simulink model "Fixed_Velocity_Fixed_Delta_TruckLab_A1"  (R2025b)
settings: Solver=ode4  StartTime=0  StopTime=130  FixedStep=1/120  RelTol=1e-3
undefined symbols (not defined in the file or in its folder): getRigidBodyPose, twist
libraries: simulink_extras x3, ros2lib x2
settings Model: Creator=20212285  LastModifiedBy=koenscholten
settings SolverCC: AlgebraicLoopSolver=LineSearch
settings DataIOCC: ReturnWorkspaceOutputsName=s
settings OptimizationCC: EnhancedBackFolding=on  PassReuseOutputArgsAs=Individual arguments  ZeroExternalMemoryAtStartup=off  ZeroInternalMemoryAtStartup=off  MaxStackSize=64  OptimizeBlockOrder=speed  DifferentSizesBufferReuse=on  OptimizationCustomize=off  EfficientTunableParamExpr=on
settings DebuggingCC: ParameterTunabilityLossMsg=error  UnconnectedInputMsg=warning  UnconnectedOutputMsg=warning  UnconnectedLineMsg=warning
settings ModelReferenceCC: EnableRefExpFcnMdlSchedulingChecks=on
settings SFSimCC: MATLABDynamicMemAlloc=off  SimTargetLang=C++  SimDLTargetLibrary=mkl-dnn
settings RTWCC: SystemTargetFile=ert.tlc  HardwareBoard=Robot Operating System 2 (ROS 2)  TLCOptions="-aInlineSetEventsForThisBaseRateFcn=TLC_FALSE -aSuppressMultiTaskScheduler=TLC_FALSE  -aRateBasedStepFcn=0"  TemplateMakefile=ert_default_tmf  Toolchain=Colcon Tools  TargetLang=C++  GPUComputeCapability=3.5  Description=Embedded Coder
settings CodeAppCC: ForceParamTrailComments=on  IgnoreCustomStorageClasses=off  OperatorAnnotations=on  SimulinkDataObjDesc=on  SFDataObjDesc=on  InsertBlockDesc=on
settings ERTTargetCC: ExtModeTransport=2.0  ExtModeStaticAlloc=on  ExtModeAutomaticAllocSize=off  ExtModeMexFile=ext_xcp  ExtModeIntrfLevel=Level2 - Open  InlinedParameterPlacement=Hierarchical  RootIOFormat=Structure reference  DynamicArrayContainerType=coder::array  CodeInterfacePackaging=C++ class

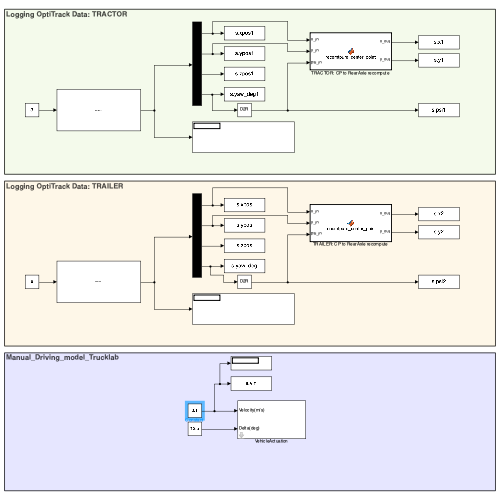
[thumbnail: Simulink's stored preview of the top-level diagram]
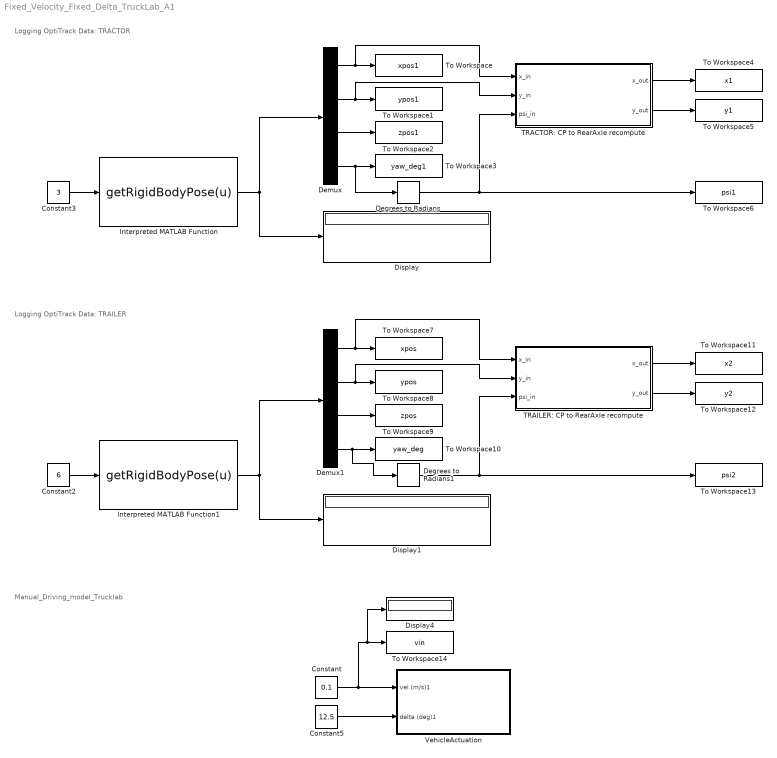
== system Fixed_Velocity_Fixed_Delta_TruckLab_A1 ==
  note: Logging OptiTrack Data: TRACTOR
  note: Manual_Driving_model_Trucklab
  note: Logging OptiTrack Data: TRAILER
  Constant : Constant  Value=0.1
  Constant2 : Constant  Value=6
  Constant3 : Constant  Value=3
  Constant5 : Constant  Value=12.5
  Degrees to Radians : simulink_extras/Transformations/Degrees to Radians
  Degrees to Radians1 : simulink_extras/Transformations/Degrees to Radians
  Demux : Demux
  Demux1 : Demux
  Display : Display
  Display1 : Display
  Display4 : Display
  Interpreted MATLAB Function : MATLABFcn  MATLABFcn=getRigidBodyPose(u)
  Interpreted MATLAB Function1 : MATLABFcn  MATLABFcn=getRigidBodyPose(u)
  TRACTOR: CP to RearAxle recompute : MATLAB Function  TreatAsAtomicUnit=on
  TRAILER: CP to RearAxle recompute : MATLAB Function  TreatAsAtomicUnit=on
  To Workspace : ToWorkspace  VariableName=xpos1  SaveFormat=Timeseries  SampleTime=-1
  To Workspace1 : ToWorkspace  VariableName=ypos1  SaveFormat=Timeseries  SampleTime=-1
  To Workspace10 : ToWorkspace  VariableName=yaw_deg  SaveFormat=Timeseries  SampleTime=-1
  To Workspace11 : ToWorkspace  VariableName=x2  SaveFormat=Timeseries  SampleTime=-1
  To Workspace12 : ToWorkspace  VariableName=y2  SaveFormat=Timeseries  SampleTime=-1
  To Workspace13 : ToWorkspace  VariableName=psi2  SaveFormat=Timeseries  SampleTime=-1
  To Workspace14 : ToWorkspace  VariableName=vin  SaveFormat=Timeseries  SampleTime=-1
  To Workspace2 : ToWorkspace  VariableName=zpos1  SaveFormat=Timeseries  SampleTime=-1
  To Workspace3 : ToWorkspace  VariableName=yaw_deg1  SaveFormat=Timeseries  SampleTime=-1
  To Workspace4 : ToWorkspace  VariableName=x1  SaveFormat=Timeseries  SampleTime=-1
  To Workspace5 : ToWorkspace  VariableName=y1  SaveFormat=Timeseries  SampleTime=-1
  To Workspace6 : ToWorkspace  VariableName=psi1  SaveFormat=Timeseries  SampleTime=-1
  To Workspace7 : ToWorkspace  VariableName=xpos  SaveFormat=Timeseries  SampleTime=-1
  To Workspace8 : ToWorkspace  VariableName=ypos  SaveFormat=Timeseries  SampleTime=-1
  To Workspace9 : ToWorkspace  VariableName=zpos  SaveFormat=Timeseries  SampleTime=-1
  VehicleActuation : Subsystem  mask(Vehicle Actuation){robotIndex=1, topic=/tractor1/cmd, messageType=geometry_msgs/Twist}
      mask prompts: robotIndex "Type the Index no."; topic "ros:slros:blockmask:TopicPrompt"; messageType "ros:slros:blockmask:MessageTypePrompt"
      mask help:
      | The velocity and steering angle inputs from the Thrustmaster Input block are published to a ROS topic. A ROS node on the actuator hardware side subscribes to this topic and executes the corresponding control actions.
      |
      | Select the tractor index that you wish to control.
      mask init:
      | % Retrieve mask parameters
      | robotIndex = str2double(get_param(gcb, 'robotIndex')); % Get the robot index
      |          % Get the topic source, if applicable
      | 
      | % Define the base path for the ROS blocks inside the subsystem
      | 
      | publishBlockPath = strcat(gcb);       % Adjust path for ROS Publish block
      | 
      | 
      | 
      | % For ROS Publish block
      | pubTopic = sprintf('/tractor%d/cmd', robotIndex);     % Example topic for Publish
      | set_param(publishBlockPath, 'Topic', pubTopic);
      | set_param(publishBlockPath, 'MessageType', 'geometry_msgs/Twist');
      mask Help:
      | Description:
      | <p style="font-family: Arial, sans-serif; font-size: 12px;"> The <b>Vehicle Actuation Block</b> provides an interface to control the physical actuators of the trucks in the <b>TruckLab</b> environment. It accepts <b>velocity (in m/s)</b> and <b>steering angle (in radians)</b> as inputs and publishes these control signals to the ROS network via the <b>ROS Publish Block</b>. </p>
      | Inputs:
      | <ul style="font-family: Arial, sans-serif; font-size: 12px;"> <li><b>Velocity (m/s):</b> Desired velocity of the truck.</li> <li><b>Steering Angle (rad):</b> Desired steering angle of the truck.</li> </ul>
      | Outputs:
      | <ul style="font-family: Arial, sans-serif; font-size: 12px;"> <li><b>ROS Message:</b> The block publishes a <b>geometry_msgs/Twist</b> message to the ROS topic <code>/tractor&lt;ID&gt;/cmd</code>, where <code>&lt;ID&gt;</code> is the truck number. The message contains: <ul> <li><b>Linear.X:</b> Velocity (m/s).</li> <li><b>Angular.Z:</b> Steering angle (rad).</li> </ul> </li> </ul>
      | Parameters:
      | <ul style="font-family: Arial, sans-serif; font-size: 12px;"> <li><b>Truck Number:</b> The ID of the truck to be controlled (e.g., 1, 2, 3). This dynamically updates the ROS topic name (e.g., <code>/tractor3/cmd</code>).</li> </ul>
      | Functionality:
      | <ol style="font-family: Arial, sans-serif; font-size: 12px;"> <li><b>Input Signals:</b> <ul> <li>The block accepts two input signals: <ul> <li><b>Velocity (m/s):</b> Controls the truck's speed.</li> <li><b>Steering Angle (rad):</b> Controls the truck's direction.</li> </ul> </li> </ul> </li> <li><b>ROS Message Setup:</b> <ul> <li>A <b>ROS Blank Message Block</b> generates a blank <b>geometry_msgs/Twist</b> message. This message type is standard for controlling mobile robots and contains two main fields: <ul> <li><b>Linear:</b> For translational motion (velocity).</li> <li><b>Angular:</b> For rotational motion (steering).</li> </ul> </li> </ul> </li> <li><b>Populating the Message:</b> <ul> <li>A <b>Bus Assignment Block</b> is used to assign the input signals to the appropriate fields in the <b>geometry_msgs/Twist</b> message: <ul> <li><b>Linear.X:</b> Assigned to the velocity input.</li> <li><b>Angular.Z:</b> Assigned to the steering angle input.</li> </ul> </li> </ul> </li> <li><b>Publishing to ROS:</b> <ul> <li>The populated message is published to the ROS topic <code>/tractor&lt;ID&gt;/cmd</code> using the <b>ROS Publish Block</b>, where <code>&lt;ID&gt;</code> is the truck number. This allows real-time control of the truck's movement.</li> </ul> </li> <li><b>Dynamic Topic Naming:</b> <ul> <li>The ROS topic name is dynamically updated based on the selected truck number (e.g., <code>/tractor3/cmd</code> for truck 3).</li> </ul> </li> </ol>
      | User Instructions:
      | <ol style="font-family: Arial, sans-serif; font-size: 12px;"> <li>Add the <b>Vehicle Actuation Block</b> to your Simulink model.</li> <li>Set the <b>Truck Number</b> parameter to match the ID of the truck you want to control.</li> <li>Connect the <b>velocity (m/s)</b> and <b>steering angle (rad)</b> signals to the block inputs.</li> <li>Run the model to publish control signals to the ROS network.</li> </ol>
      | Example Usage:
      | <p style="font-family: Arial, sans-serif; font-size: 12px;"> To control <b>Tractor 3</b>, set the <b>Truck Number</b> to 3. The block will publish velocity and steering angle commands to the ROS topic <code>/tractor3/cmd</code>. </p>
      | References:
      | <ul style="font-family: Arial, sans-serif; font-size: 12px;"> <li><b>ROS Publish Block Documentation:</b> <a href="https://nl.mathworks.com/help/ros/ref/publish.html">https://nl.mathworks.com/help/ros/ref/publish.html</a></li> <li><b>ROS Blank Message Block Documentation:</b> <a href="https://nl.mathworks.com/help/ros/ref/blankmessage.html">https://nl.mathworks.com/help/ros/ref/blankmessage.html</a></li> </ul>
      mask TypeOptions topic: Publish1/topic
      mask TypeOptions messageType: Publish1/messageType
      mask DialogControl topic Prompt: Topic:
      mask DialogControl messageType Prompt: Message type:
      mask Display:
      | port_label('input', 1, 'Velocity(m/s)')
      | port_label('input', 2, 'Delta(deg)')
  wires:
  Constant/1 -> Display4/1, To Workspace14/1, VehicleActuation/1(vel (m/s)1)
  Demux/4 -> Degrees to Radians/1, To Workspace3/1
  Interpreted MATLAB Function/1 -> Display/1, Demux/1
  Demux/1 -> To Workspace/1, TRACTOR: CP to RearAxle recompute/1(x_in)
  Demux/2 -> TRACTOR: CP to RearAxle recompute/2(y_in), To Workspace1/1
  Demux/3 -> To Workspace2/1
  Degrees to Radians/1 -> To Workspace6/1, TRACTOR: CP to RearAxle recompute/3(psi_in)
  TRACTOR: CP to RearAxle recompute/1(x_out) -> To Workspace4/1
  TRACTOR: CP to RearAxle recompute/2(y_out) -> To Workspace5/1
  TRAILER: CP to RearAxle recompute/1(x_out) -> To Workspace11/1
  Degrees to Radians1/1 -> To Workspace13/1, TRAILER: CP to RearAxle recompute/3(psi_in)
  TRAILER: CP to RearAxle recompute/2(y_out) -> To Workspace12/1
  Demux1/1 -> To Workspace7/1, TRAILER: CP to RearAxle recompute/1(x_in)
  Demux1/2 -> TRAILER: CP to RearAxle recompute/2(y_in), To Workspace8/1
  Demux1/4 -> Degrees to Radians1/1, To Workspace10/1
  Demux1/3 -> To Workspace9/1
  Interpreted MATLAB Function1/1 -> Display1/1, Demux1/1
  Constant2/1 -> Interpreted MATLAB Function1/1
  Constant3/1 -> Interpreted MATLAB Function/1
  Constant5/1 -> VehicleActuation/2(delta (deg)1)

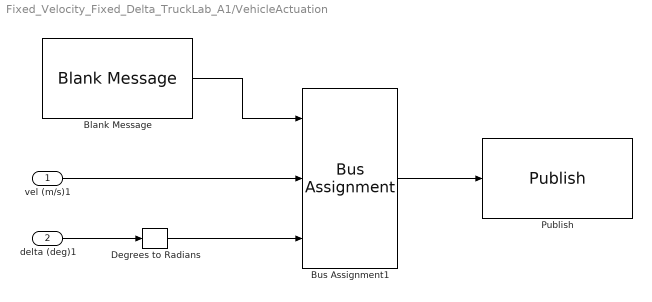
== system Fixed_Velocity_Fixed_Delta_TruckLab_A1/VehicleActuation ==
  vel (m/s)1 : Inport
  delta (deg)1 : Inport  Port=2
  Blank Message : ros2lib/Blank Message  messageClass=Message  entityType=geometry_msgs/TwistStamped  messageType=geometry_msgs/TwistStamped  SampleTime=1/120
  Bus Assignment1 : BusAssignment  DialogController=Simulink.DDGSource_BusAssignment  AssignedSignals=twist.linear.x,twist.angular.z
  Degrees to Radians : simulink_extras/Transformations/Degrees to Radians
  Publish : ros2lib/Publish  topicSource=Select from ROS network  topic=/tractor3/cmd_vel  messageType=geometry_msgs/TwistStamped  QOSHistory=Keep last  QOSDepth=10  QOSReliability=Reliable  QOSDurability=Volatile  QOSDeadline=Inf  QOSLifespan=Inf  QOSLiveliness=Automatic  QOSLeaseDuration=Inf  QOSAvoidROSNamespaceConventions=off
  wires:
  Bus Assignment1/1 -> Publish/1
  delta (deg)1/1 -> Degrees to Radians/1
  vel (m/s)1/1 -> Bus Assignment1/2
  Degrees to Radians/1 -> Bus Assignment1/3
  Blank Message/1 -> Bus Assignment1/1

== matlab function Fixed_Velocity_Fixed_Delta_TruckLab_A1/TRAILER: CP to RearAxle recompute ==
  data: x_in input; y_in input; psi_in input; x_out output; y_out output
function [x_out, y_out] = recomtpure_center_point(x_in, y_in, psi_in)

    cp_offset = 0.18; %[m]

    x_out = x_in - cp_offset*cos(psi_in);
    y_out = y_in - cp_offset*sin(psi_in);

== matlab function Fixed_Velocity_Fixed_Delta_TruckLab_A1/TRACTOR: CP to RearAxle recompute ==
  data: x_in input; y_in input; psi_in input; x_out output; y_out output
function [x_out, y_out] = recomtpure_center_point(x_in, y_in, psi_in)

    cp_offset = 0.31; %[m]

    x_out = x_in - cp_offset*cos(psi_in);
    y_out = y_in - cp_offset*sin(psi_in);
